simulink model "LedCount_load"  (R2014a)
settings: Solver=FixedStepDiscrete  StartTime=0.0  StopTime=400000  FixedStep=1  RelTol=1e-3
libraries: hdlsllib x19, simulink x6
settings Model: Creator=you.r  LastModifiedBy=you.r
settings OptimizationCC: BlockReduction=off  ConditionallyExecuteInputs=off  InlineParams=on
settings DebuggingCC: AlgebraicLoopMsg=error
settings HardwareCC: ProdHWDeviceType=ASIC/FPGA->ASIC/FPGA  ProdEqTarget=off

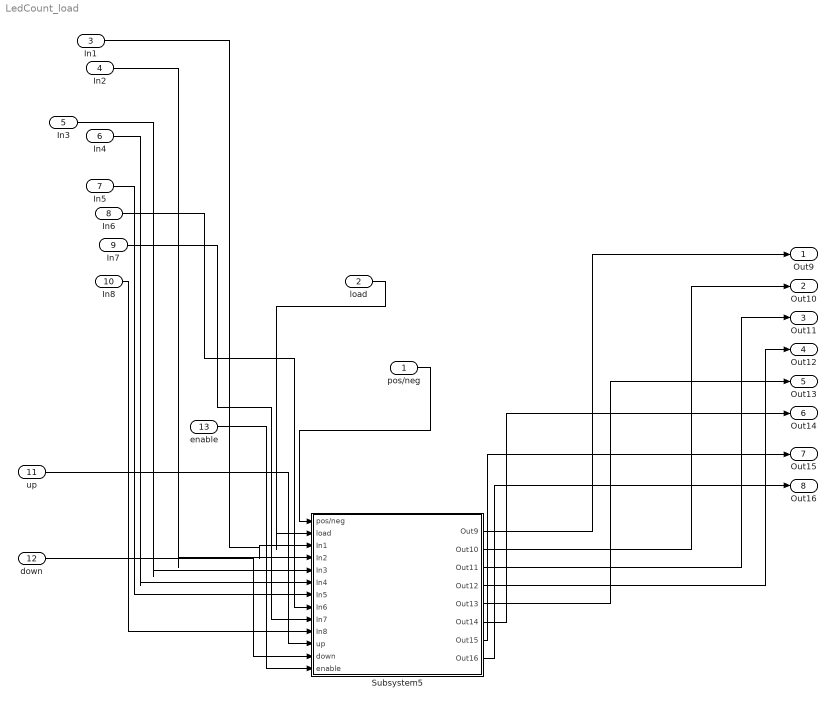
== system LedCount_load ==
  pos/neg : Inport  OutDataTypeStr=boolean  SampleTime=1
  load : Inport  Port=2  OutDataTypeStr=boolean  SampleTime=1
  In1 : Inport  Port=3
  In2 : Inport  Port=4
  In3 : Inport  Port=5
  In4 : Inport  Port=6
  In5 : Inport  Port=7
  In6 : Inport  Port=8
  In7 : Inport  Port=9
  In8 : Inport  Port=10
  up : Inport  Port=11  OutDataTypeStr=boolean  SampleTime=1
  down : Inport  Port=12  OutDataTypeStr=boolean  SampleTime=1
  enable : Inport  Port=13  OutDataTypeStr=boolean  SampleTime=1
  Subsystem5 : Subsystem  TreatAsAtomicUnit=on
  Out9 : Outport  SampleTime=1
  Out10 : Outport  Port=2  SampleTime=1
  Out11 : Outport  Port=3  SampleTime=1
  Out12 : Outport  Port=4  SampleTime=1
  Out13 : Outport  Port=5  SampleTime=1
  Out14 : Outport  Port=6  SampleTime=1
  Out15 : Outport  Port=7  SampleTime=1
  Out16 : Outport  Port=8  SampleTime=1
  wires:
  pos/neg/1 -> Subsystem5/1(pos/neg)
  load/1 -> Subsystem5/2(load)
  In1/1 -> Subsystem5/3(In1)
  In2/1 -> Subsystem5/4(In2)
  In3/1 -> Subsystem5/5(In3)
  In4/1 -> Subsystem5/6(In4)
  In5/1 -> Subsystem5/7(In5)
  In6/1 -> Subsystem5/8(In6)
  In7/1 -> Subsystem5/9(In7)
  In8/1 -> Subsystem5/10(In8)
  up/1 -> Subsystem5/11(up)
  down/1 -> Subsystem5/12(down)
  enable/1 -> Subsystem5/13(enable)
  Subsystem5/1(Out9) -> Out9/1
  Subsystem5/2(Out10) -> Out10/1
  Subsystem5/3(Out11) -> Out11/1
  Subsystem5/4(Out12) -> Out12/1
  Subsystem5/5(Out13) -> Out13/1
  Subsystem5/6(Out14) -> Out14/1
  Subsystem5/7(Out15) -> Out15/1
  Subsystem5/8(Out16) -> Out16/1

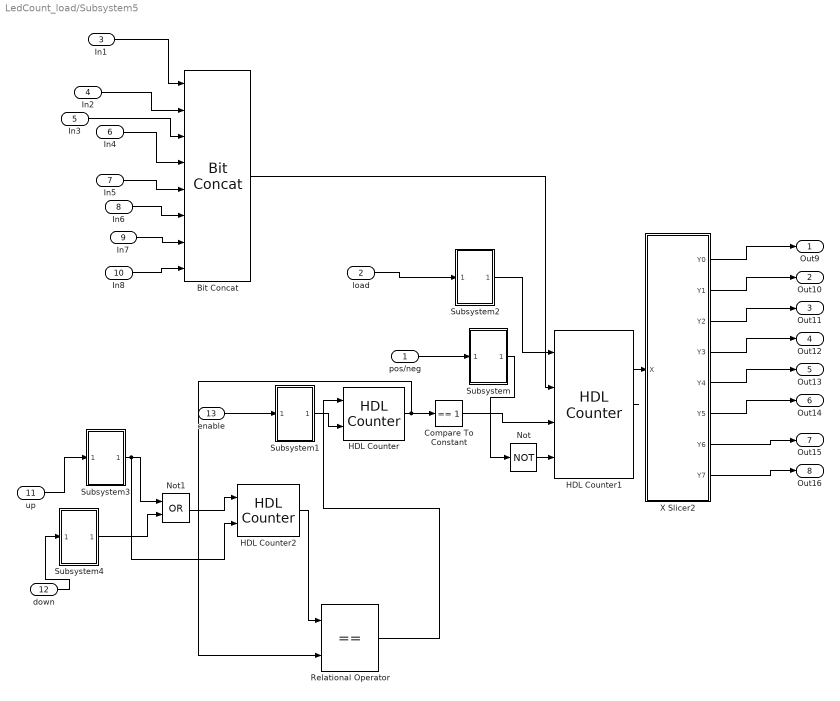
== system LedCount_load/Subsystem5 ==
  pos/neg : Inport  OutDataTypeStr=boolean  SampleTime=1
  load : Inport  Port=2  OutDataTypeStr=boolean  SampleTime=1
  In1 : Inport  Port=3  OutDataTypeStr=boolean  SampleTime=1
  In2 : Inport  Port=4  OutDataTypeStr=boolean  SampleTime=1
  In3 : Inport  Port=5  OutDataTypeStr=boolean  SampleTime=1
  In4 : Inport  Port=6  OutDataTypeStr=boolean  SampleTime=1
  In5 : Inport  Port=7  OutDataTypeStr=boolean  SampleTime=1
  In6 : Inport  Port=8  OutDataTypeStr=boolean  SampleTime=1
  In7 : Inport  Port=9  OutDataTypeStr=boolean  SampleTime=1
  In8 : Inport  Port=10  OutDataTypeStr=boolean  SampleTime=1
  up : Inport  Port=11  OutDataTypeStr=boolean  SampleTime=1
  down : Inport  Port=12  OutDataTypeStr=boolean  SampleTime=1
  enable : Inport  Port=13  OutDataTypeStr=boolean  SampleTime=1
  Bit Concat : hdlsllib/HDL Operations/Bit Concat  numInputs=8
  Compare To Constant : simulink/Logic and Bit Operations/Compare To Constant  relop===  const=1  OutDataTypeStr=boolean
  HDL Counter : hdlsllib/HDL Operations/HDL Counter  CountType=Count limited  CountInit=100000  CountStep=100000  CountMax=100000000  CountFromType=Initial value  CountFrom=100000  CountResetPort=on  CountLoadPort=off  CountEnbPort=on  CountDirPort=off  CountDataType=Unsigned  CountWordLen=32  CountFracLen=0  CountSampTime=1
  HDL Counter1 : hdlsllib/HDL Operations/HDL Counter  CountType=Count limited  CountInit=0  CountStep=1  CountMax=255  CountFromType=Initial value  CountFrom=0  CountResetPort=off  CountLoadPort=on  CountEnbPort=on  CountDirPort=on  CountDataType=Unsigned  CountWordLen=8  CountFracLen=0  CountSampTime=1
  HDL Counter2 : hdlsllib/HDL Operations/HDL Counter  CountType=Count limited  CountInit=20000000  CountStep=1000000  CountMax=100000000  CountFromType=Initial value  CountFrom=20000000  CountResetPort=off  CountLoadPort=off  CountEnbPort=on  CountDirPort=on  CountDataType=Unsigned  CountWordLen=32  CountFracLen=0  CountSampTime=1
  Not : Logic  Operator=NOT  AllPortsSameDT=off  OutDataTypeStr=boolean
  Not1 : Logic  Operator=OR  AllPortsSameDT=off  OutDataTypeStr=boolean
  Relational Operator : RelationalOperator  Operator===  OutDataTypeStr=boolean  SampleTime=1
  Subsystem : Subsystem
  Subsystem1 : Subsystem
  Subsystem2 : Subsystem
  Subsystem3 : Subsystem
  Subsystem4 : Subsystem
  X Slicer2 : Subsystem
  Out9 : Outport  SampleTime=1
  Out10 : Outport  Port=2  SampleTime=1
  Out11 : Outport  Port=3  SampleTime=1
  Out12 : Outport  Port=4  SampleTime=1
  Out13 : Outport  Port=5  SampleTime=1
  Out14 : Outport  Port=6  SampleTime=1
  Out15 : Outport  Port=7  SampleTime=1
  Out16 : Outport  Port=8  SampleTime=1
  wires:
  HDL Counter/1 -> Relational Operator/2, Compare To Constant/1
  HDL Counter2/1 -> Relational Operator/1
  Bit Concat/1 -> HDL Counter1/2
  X Slicer2/8(Y7) -> Out16/1
  X Slicer2/1(Y0) -> Out9/1
  X Slicer2/3(Y2) -> Out11/1
  X Slicer2/5(Y4) -> Out13/1
  X Slicer2/4(Y3) -> Out12/1
  pos/neg/1 -> Subsystem/1(In1)
  Subsystem/1(Out1) -> Not/1
  X Slicer2/7(Y6) -> Out15/1
  X Slicer2/2(Y1) -> Out10/1
  X Slicer2/6(Y5) -> Out14/1
  HDL Counter1/1 -> X Slicer2/1(X)
  In7/1 -> Bit Concat/7
  In6/1 -> Bit Concat/6
  In2/1 -> Bit Concat/2
  In1/1 -> Bit Concat/1
  In3/1 -> Bit Concat/3
  In4/1 -> Bit Concat/4
  In5/1 -> Bit Concat/5
  In8/1 -> Bit Concat/8
  down/1 -> Subsystem4/1(In1)
  up/1 -> Subsystem3/1(In1)
  Subsystem4/1(Out1) -> Not1/2
  Not1/1 -> HDL Counter2/1
  Not/1 -> HDL Counter1/4
  enable/1 -> Subsystem1/1(In1)
  Subsystem3/1(Out1) -> Not1/1, HDL Counter2/2
  load/1 -> Subsystem2/1(In1)
  Subsystem2/1(Out1) -> HDL Counter1/1
  Compare To Constant/1 -> HDL Counter1/3
  Relational Operator/1 -> HDL Counter/1
  Subsystem1/1(Out1) -> HDL Counter/2

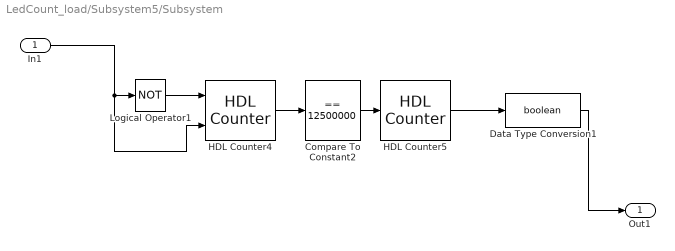
== system LedCount_load/Subsystem5/Subsystem ==
  In1 : Inport
  Compare To Constant2 : simulink/Logic and Bit Operations/Compare To Constant  relop===  const=12500000  OutDataTypeStr=boolean
  Data Type Conversion1 : DataTypeConversion  OutDataTypeStr=boolean
  HDL Counter4 : hdlsllib/HDL Operations/HDL Counter  CountType=Free running  CountInit=0  CountStep=1  CountMax=100  CountFromType=Initial value  CountFrom=0  CountResetPort=on  CountLoadPort=off  CountEnbPort=on  CountDirPort=off  CountDataType=Unsigned  CountWordLen=32  CountFracLen=0  CountSampTime=1
  HDL Counter5 : hdlsllib/HDL Operations/HDL Counter  CountType=Count limited  CountInit=0  CountStep=1  CountMax=1  CountFromType=Initial value  CountFrom=0  CountResetPort=off  CountLoadPort=off  CountEnbPort=on  CountDirPort=off  CountDataType=Unsigned  CountWordLen=1  CountFracLen=0  CountSampTime=1
  Logical Operator1 : Logic  Operator=NOT  IconShape=distinctive  AllPortsSameDT=off  OutDataTypeStr=boolean  SampleTime=1
  Out1 : Outport
  wires:
  Compare To Constant2/1 -> HDL Counter5/1
  Logical Operator1/1 -> HDL Counter4/1
  HDL Counter5/1 -> Data Type Conversion1/1
  In1/1 -> HDL Counter4/2, Logical Operator1/1
  Data Type Conversion1/1 -> Out1/1
  HDL Counter4/1 -> Compare To Constant2/1

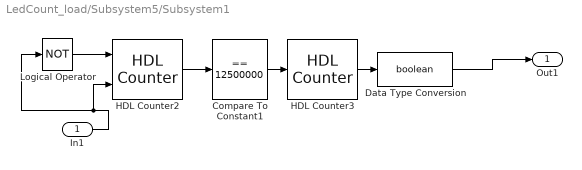
== system LedCount_load/Subsystem5/Subsystem1 ==
  In1 : Inport
  Compare To Constant1 : simulink/Logic and Bit Operations/Compare To Constant  relop===  const=12500000  OutDataTypeStr=boolean
  Data Type Conversion : DataTypeConversion  OutDataTypeStr=boolean
  HDL Counter2 : hdlsllib/HDL Operations/HDL Counter  CountType=Free running  CountInit=0  CountStep=1  CountMax=100  CountFromType=Initial value  CountFrom=0  CountResetPort=on  CountLoadPort=off  CountEnbPort=on  CountDirPort=off  CountDataType=Unsigned  CountWordLen=32  CountFracLen=0  CountSampTime=1
  HDL Counter3 : hdlsllib/HDL Operations/HDL Counter  CountType=Count limited  CountInit=0  CountStep=1  CountMax=1  CountFromType=Initial value  CountFrom=0  CountResetPort=off  CountLoadPort=off  CountEnbPort=on  CountDirPort=off  CountDataType=Unsigned  CountWordLen=1  CountFracLen=0  CountSampTime=1
  Logical Operator : Logic  Operator=NOT  IconShape=distinctive  AllPortsSameDT=off  OutDataTypeStr=boolean  SampleTime=1
  Out1 : Outport
  wires:
  HDL Counter2/1 -> Compare To Constant1/1
  Logical Operator/1 -> HDL Counter2/1
  In1/1 -> Logical Operator/1, HDL Counter2/2
  Data Type Conversion/1 -> Out1/1
  HDL Counter3/1 -> Data Type Conversion/1
  Compare To Constant1/1 -> HDL Counter3/1

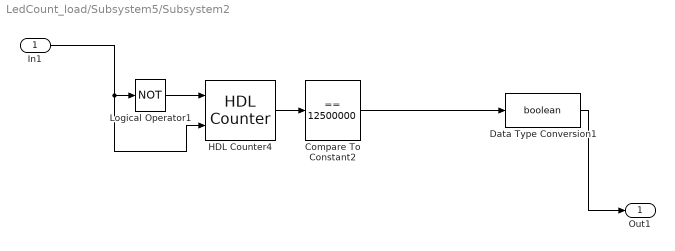
== system LedCount_load/Subsystem5/Subsystem2 ==
  In1 : Inport
  Compare To Constant2 : simulink/Logic and Bit Operations/Compare To Constant  relop===  const=12500000  OutDataTypeStr=boolean
  Data Type Conversion1 : DataTypeConversion  OutDataTypeStr=boolean
  HDL Counter4 : hdlsllib/HDL Operations/HDL Counter  CountType=Free running  CountInit=0  CountStep=1  CountMax=100  CountFromType=Initial value  CountFrom=0  CountResetPort=on  CountLoadPort=off  CountEnbPort=on  CountDirPort=off  CountDataType=Unsigned  CountWordLen=32  CountFracLen=0  CountSampTime=1
  Logical Operator1 : Logic  Operator=NOT  IconShape=distinctive  AllPortsSameDT=off  OutDataTypeStr=boolean  SampleTime=1
  Out1 : Outport
  wires:
  Logical Operator1/1 -> HDL Counter4/1
  Compare To Constant2/1 -> Data Type Conversion1/1
  In1/1 -> HDL Counter4/2, Logical Operator1/1
  Data Type Conversion1/1 -> Out1/1
  HDL Counter4/1 -> Compare To Constant2/1

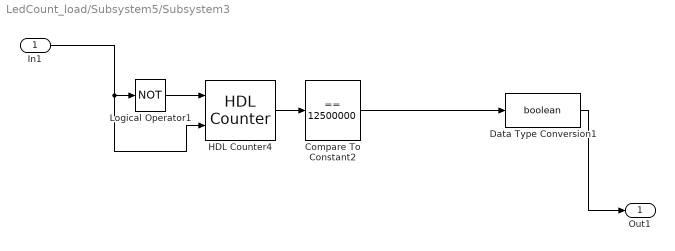
== system LedCount_load/Subsystem5/Subsystem3 ==
  In1 : Inport
  Compare To Constant2 : simulink/Logic and Bit Operations/Compare To Constant  relop===  const=12500000  OutDataTypeStr=boolean
  Data Type Conversion1 : DataTypeConversion  OutDataTypeStr=boolean
  HDL Counter4 : hdlsllib/HDL Operations/HDL Counter  CountType=Free running  CountInit=0  CountStep=1  CountMax=100  CountFromType=Initial value  CountFrom=0  CountResetPort=on  CountLoadPort=off  CountEnbPort=on  CountDirPort=off  CountDataType=Unsigned  CountWordLen=32  CountFracLen=0  CountSampTime=1
  Logical Operator1 : Logic  Operator=NOT  IconShape=distinctive  AllPortsSameDT=off  OutDataTypeStr=boolean  SampleTime=1
  Out1 : Outport
  wires:
  Logical Operator1/1 -> HDL Counter4/1
  Compare To Constant2/1 -> Data Type Conversion1/1
  In1/1 -> HDL Counter4/2, Logical Operator1/1
  Data Type Conversion1/1 -> Out1/1
  HDL Counter4/1 -> Compare To Constant2/1

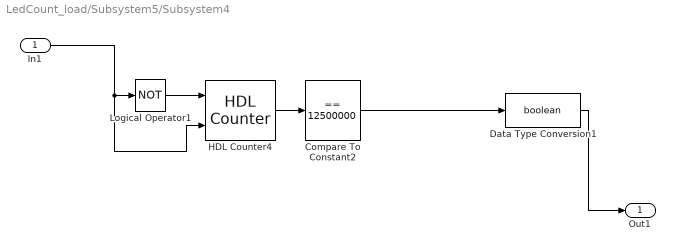
== system LedCount_load/Subsystem5/Subsystem4 ==
  In1 : Inport
  Compare To Constant2 : simulink/Logic and Bit Operations/Compare To Constant  relop===  const=12500000  OutDataTypeStr=boolean
  Data Type Conversion1 : DataTypeConversion  OutDataTypeStr=boolean
  HDL Counter4 : hdlsllib/HDL Operations/HDL Counter  CountType=Free running  CountInit=0  CountStep=1  CountMax=100  CountFromType=Initial value  CountFrom=0  CountResetPort=on  CountLoadPort=off  CountEnbPort=on  CountDirPort=off  CountDataType=Unsigned  CountWordLen=32  CountFracLen=0  CountSampTime=1
  Logical Operator1 : Logic  Operator=NOT  IconShape=distinctive  AllPortsSameDT=off  OutDataTypeStr=boolean  SampleTime=1
  Out1 : Outport
  wires:
  Logical Operator1/1 -> HDL Counter4/1
  Compare To Constant2/1 -> Data Type Conversion1/1
  In1/1 -> HDL Counter4/2, Logical Operator1/1
  Data Type Conversion1/1 -> Out1/1
  HDL Counter4/1 -> Compare To Constant2/1

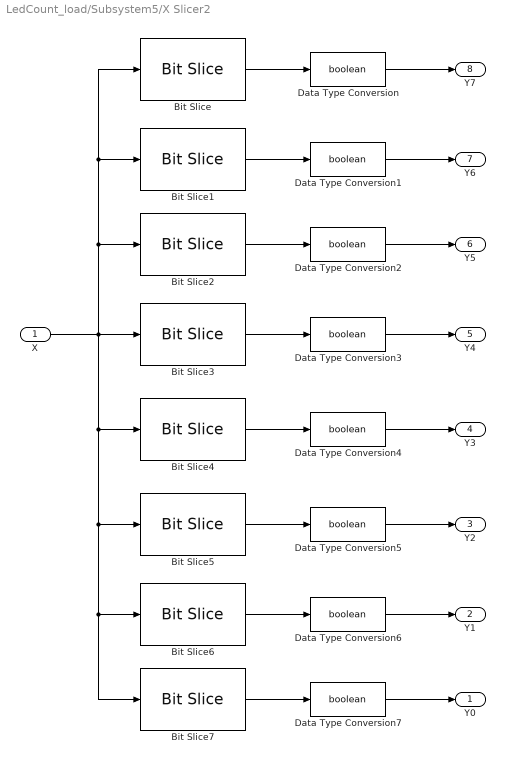
== system LedCount_load/Subsystem5/X Slicer2 ==
  X : Inport  OutDataTypeStr=uint8  SampleTime=1
  Bit Slice : hdlsllib/HDL Operations/Bit Slice  lidx=7  ridx=7
  Bit Slice1 : hdlsllib/HDL Operations/Bit Slice  lidx=6  ridx=6
  Bit Slice2 : hdlsllib/HDL Operations/Bit Slice  lidx=5  ridx=5
  Bit Slice3 : hdlsllib/HDL Operations/Bit Slice  lidx=4  ridx=4
  Bit Slice4 : hdlsllib/HDL Operations/Bit Slice  lidx=3  ridx=3
  Bit Slice5 : hdlsllib/HDL Operations/Bit Slice  lidx=2  ridx=2
  Bit Slice6 : hdlsllib/HDL Operations/Bit Slice  lidx=1  ridx=1
  Bit Slice7 : hdlsllib/HDL Operations/Bit Slice  lidx=0  ridx=0
  Data Type Conversion{,1..7} (8 alike) : DataTypeConversion  OutDataTypeStr=boolean
  Y0 : Outport  OutDataTypeStr=boolean  SampleTime=1
  Y1 : Outport  Port=2  OutDataTypeStr=boolean  SampleTime=1
  Y2 : Outport  Port=3  OutDataTypeStr=boolean  SampleTime=1
  Y3 : Outport  Port=4  OutDataTypeStr=boolean  SampleTime=1
  Y4 : Outport  Port=5  OutDataTypeStr=boolean  SampleTime=1
  Y5 : Outport  Port=6  OutDataTypeStr=boolean  SampleTime=1
  Y6 : Outport  Port=7  OutDataTypeStr=boolean  SampleTime=1
  Y7 : Outport  Port=8  OutDataTypeStr=boolean  SampleTime=1
  wires:
  X/1 -> Bit Slice4/1, Bit Slice5/1, Bit Slice6/1, Bit Slice7/1, Bit Slice3/1, Bit Slice2/1, Bit Slice1/1, Bit Slice/1
  Data Type Conversion/1 -> Y7/1
  Data Type Conversion1/1 -> Y6/1
  Bit Slice2/1 -> Data Type Conversion2/1
  Bit Slice3/1 -> Data Type Conversion3/1
  Bit Slice4/1 -> Data Type Conversion4/1
  Data Type Conversion6/1 -> Y1/1
  Bit Slice/1 -> Data Type Conversion/1
  Bit Slice1/1 -> Data Type Conversion1/1
  Bit Slice6/1 -> Data Type Conversion6/1
  Data Type Conversion7/1 -> Y0/1
  Bit Slice7/1 -> Data Type Conversion7/1
  Bit Slice5/1 -> Data Type Conversion5/1
  Data Type Conversion2/1 -> Y5/1
  Data Type Conversion3/1 -> Y4/1
  Data Type Conversion4/1 -> Y3/1
  Data Type Conversion5/1 -> Y2/1
